simulink model "plant_linear"  (R2018a)
settings: Solver=VariableStepAuto  StartTime=0.0  StopTime=30  RelTol=1e-3
InitFcn:
  | kf = 10;
  | m = 0.1;
  | c = 3;
  | k = 10;
  | 
  | b3 = m;
  | b2 = 0.1;
  | b1 = 1.0;
  | b0 = 4;
settings Model: Creator=saad  LastModifiedBy=saad
settings HardwareCC: ProdBitPerLong=64  ProdHWDeviceType=Intel->x86-64 (Linux 64)  TargetBitPerLong=64  TargetBitPerPointer=64  TargetBitPerSizeT=64  TargetBitPerPtrDiffT=64  TargetLongLongMode=on  TargetIntDivRoundTo=Zero  TargetEndianess=LittleEndian  TargetWordSize=64  TargetHWDeviceType=Custom Processor->MATLAB Host Computer  ProdEqTarget=off

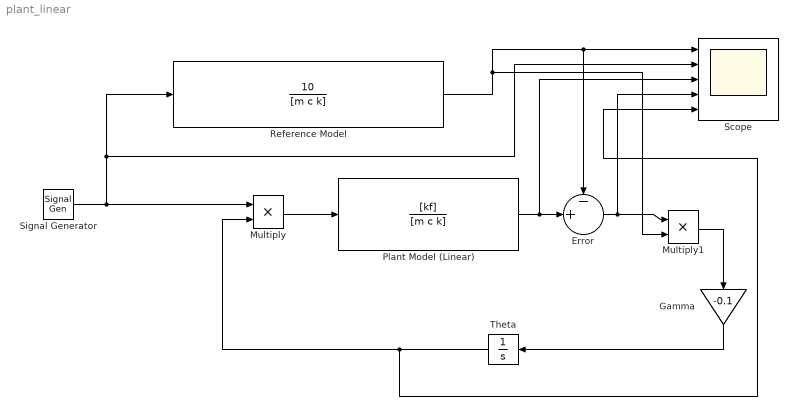
== system plant_linear ==
  Error : Sum  Inputs=-+|
  Gamma : Gain  Gain=-0.1
  Multiply : Product
  Multiply1 : Product
  Plant Model (Linear) : TransferFcn  Numerator=[kf]  Denominator=[m c k]
  Reference Model : TransferFcn  Numerator=[10]  Denominator=[m c k]
  Scope : Scope  NumInputPorts=5
  Signal Generator : SignalGenerator  WaveForm=square  Amplitude=10  Frequency=0.1
  Theta : Integrator
  wires:
  Multiply/1 -> Plant Model (Linear)/1
  Signal Generator/1 -> Multiply/1, Reference Model/1, Scope/2
  Plant Model (Linear)/1 -> Scope/3, Error/2
  Reference Model/1 -> Scope/1, Error/1, Multiply1/2
  Error/1 -> Scope/4, Multiply1/1
  Multiply1/1 -> Gamma/1
  Gamma/1 -> Theta/1
  Theta/1 -> Scope/5, Multiply/2
